simulink model "Motores"  (R2023b)
settings: Solver=FixedStepAuto  StartTime=0.0  StopTime=inf  RelTol=1e-3  EnableMultiTasking=on
libraries: arduinolib x6
settings Model: ExtModeTrigDuration=2  Creator=Manuel  LastModifiedBy=Manuel
settings OptimizationCC: EnhancedBackFolding=on  PassReuseOutputArgsAs=Individual arguments  ZeroExternalMemoryAtStartup=off  ZeroInternalMemoryAtStartup=off  MaxStackSize=64  OptimizeBlockOrder=speed  DifferentSizesBufferReuse=on  OptimizationCustomize=off  EfficientTunableParamExpr=on
settings DebuggingCC: ParameterTunabilityLossMsg=error
settings HardwareCC: ProdBitPerInt=16  ProdBitPerPointer=16  ProdBitPerSizeT=16  ProdBitPerPtrDiffT=16  ProdLargestAtomicFloat=None  ProdWordSize=8  ProdHWDeviceType=Atmel->AVR
settings SFSimCC: MATLABDynamicMemAlloc=off
settings RTWCC: Description=Embedded Coder  SystemTargetFile=ert.tlc  HardwareBoard=Arduino Mega 2560  TemplateMakefile=ert_default_tmf  Toolchain=Arduino AVR  BuildConfiguration=Faster Runs
settings CodeAppCC: ForceParamTrailComments=on  IgnoreCustomStorageClasses=off  OperatorAnnotations=on  SimulinkDataObjDesc=on  SFDataObjDesc=on  InsertBlockDesc=on
settings ERTTargetCC: SupportContinuousTime=on  SupportVariableSizeSignals=on  ExtModeTransport=3  ExtModeStaticAlloc=on  ExtModeAutomaticAllocSize=off  ExtModeStaticAllocSize=2048  ExtModeMexFile=ext_xcp  ExtModeIntrfLevel=Level2 - Open

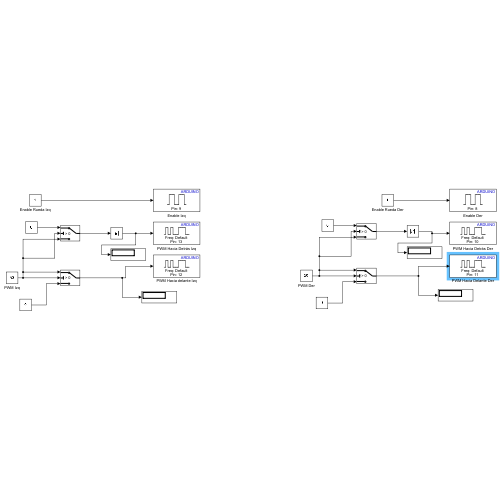
[thumbnail: Simulink's stored preview of the top-level diagram]
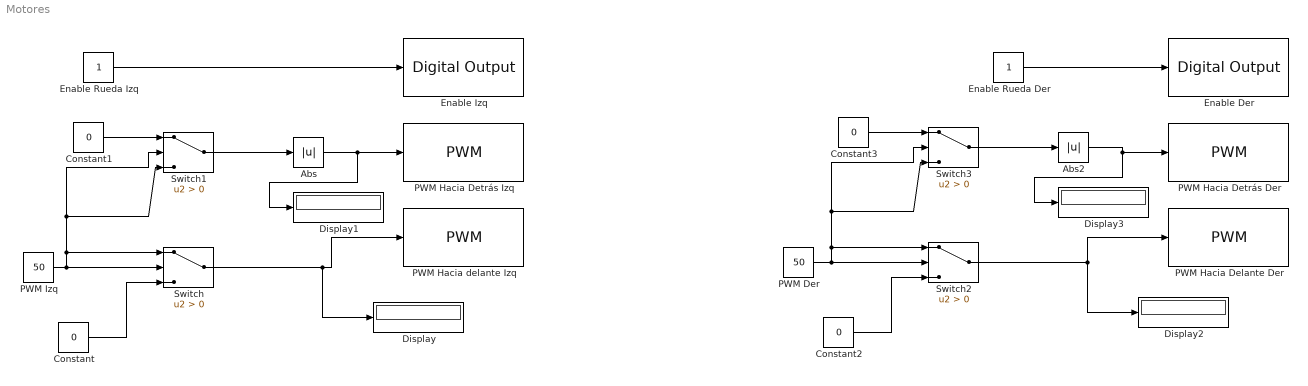
== system Motores ==
  Abs : Abs  SaturateOnIntegerOverflow=off
  Abs2 : Abs  SaturateOnIntegerOverflow=off
  Constant{,1..3} (4 alike) : Constant  Value=0
  Display{,1..3} (4 alike) : Display
  Enable Der : arduinolib/Digital Output  pinNumber=8  Direction=output  blockPlatform=arduino
  Enable Izq : arduinolib/Digital Output  pinNumber=9  Direction=output  blockPlatform=arduino
  Enable Rueda Der : Constant
  Enable Rueda Izq : Constant
  PWM Der : Constant  Value=50
  PWM Hacia Delante Der : arduinolib/PWM  pinNumber=11  frequencyType=Default  desiredFrequency=490.2  achievableFrequency=490.2
  PWM Hacia Detrás Der : arduinolib/PWM  pinNumber=10  frequencyType=Default  desiredFrequency=490.2  achievableFrequency=490.2
  PWM Hacia Detrás Izq : arduinolib/PWM  pinNumber=13  frequencyType=Default  desiredFrequency=490.2  achievableFrequency=490.2
  PWM Hacia delante Izq : arduinolib/PWM  pinNumber=12  frequencyType=Default  desiredFrequency=490.2  achievableFrequency=490.2
  PWM Izq : Constant  Value=50
  Switch{,1..3} (4 alike) : Switch  Criteria=u2 > Threshold  SaturateOnIntegerOverflow=off  InputSameDT=off
  wires:
  Enable Rueda Izq/1 -> Enable Izq/1
  Enable Rueda Der/1 -> Enable Der/1
  Abs/1 -> Display1/1, PWM Hacia Detrás Izq/1
  Switch/1 -> Display/1, PWM Hacia delante Izq/1
  PWM Izq/1 -> Switch1/2, Switch1/3, Switch/1, Switch/2
  Constant/1 -> Switch/3
  Switch1/1 -> Abs/1
  Constant1/1 -> Switch1/1
  Constant3/1 -> Switch3/1
  Abs2/1 -> PWM Hacia Detrás Der/1, Display3/1
  Switch3/1 -> Abs2/1
  Constant2/1 -> Switch2/3
  Switch2/1 -> PWM Hacia Delante Der/1, Display2/1
  PWM Der/1 -> Switch3/2, Switch3/3, Switch2/1, Switch2/2
